simulink model "SprungartigesOeffnen"  (R2018b)
settings: Solver=ode45  StartTime=0.0  StopTime=10  MaxStep=0.02  RelTol=1e-3  EnableMultiTasking=on
model workspace (MAT data in the model file):
  AFS = 30
  AS = 0.5
settings Model: Creator=Reichl  LastModifiedBy=Reichl
settings DataIOCC: SaveFormat=Array  OutputSaveName=h
settings OptimizationCC: LifeSpan=inf
settings DebuggingCC: SolverPrmCheckMsg=warning  SFUnexpectedBacktrackingDiag=warning  SFNoUnconditionalDefaultTransitionDiag=warning  SFExecutionAtInitializationDiag=none
settings HardwareCC: ProdBitPerPointer=32  ProdBitPerSizeT=32  ProdBitPerPtrDiffT=32  ProdLargestAtomicFloat=None  ProdIntDivRoundTo=Undefined  ProdEndianess=Unspecified  ProdWordSize=32  ProdHWDeviceType=32-bit Generic
settings ModelReferenceCC: PropagateSignalLabelsOutOfModel=off
settings SFSimCC: SimUseLocalCustomCode=off
settings RTWCC: RTWUseLocalCustomCode=off
settings CodeAppCC: StateflowObjectComments=on
settings GRTTargetCC: TargetLangStandard=C89/C90 (ANSI)  GeneratePreprocessorConditionals=Disable all
settings ConfigComp: CovMetricSettings=dw  CovHtmlReporting=on  CovSaveCumulativeToWorkspaceVar=on  CovSaveSingleToWorkspaceVar=on  CovExternalEMLEnable=off  CovSFcnEnable=off

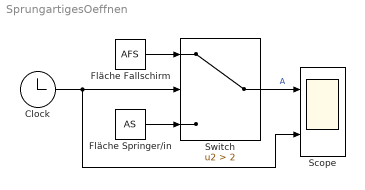
== system SprungartigesOeffnen ==
  Clock : Clock
  Fläche Fallschirm : Constant  Value=AFS
  Fläche Springer/in : Constant  Value=AS
  Scope : Scope  NumInputPorts=2
  Switch : Switch  Criteria=u2 > Threshold  Threshold=2  ZeroCross=off
  wires:
  Switch/1 -> Scope/1  "A"
  Clock/1 -> Scope/2, Switch/2
  Fläche Fallschirm/1 -> Switch/1
  Fläche Springer/in/1 -> Switch/3
